simulink model "step_down_chopper"  (R2019b)
settings: Solver=VariableStepAuto  StartTime=0.0  StopTime=0.01  RelTol=1e-3
libraries: powerlib x9, powerlib_meascontrol x1
settings Model: Creator=DELL  LastModifiedBy=DELL

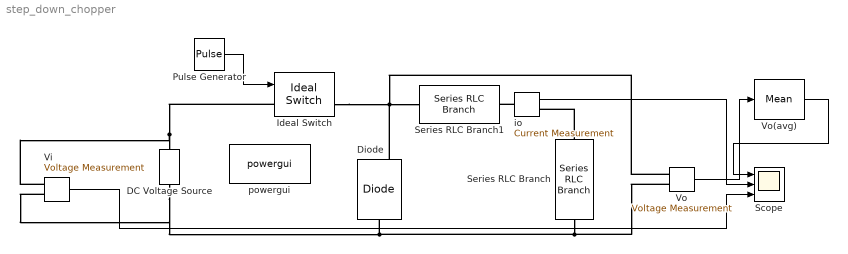
== system step_down_chopper ==
  DC Voltage Source : powerlib/Electrical Sources/DC Voltage Source  Amplitude=200  Measurements=Voltage
      settings: SourceProductName=Simscape Electrical
  Diode : powerlib/Power Electronics/Diode  Ron=0.001  Lon=0  Vf=0.8  IC=0  UseSnubber=0  Rs=500  Cs=250e-9  Measurements=on
      settings: SourceProductName=Simscape Electrical
  Ideal Switch : powerlib/Power Electronics/Ideal Switch  Ron=0.001  Lon=0  IC=0  Rs=1e5  Cs=inf  Measurements=on
      settings: SourceProductName=Simscape Electrical
  Pulse Generator : DiscretePulseGenerator  PulseType=Time based  Period=0.001  PulseWidth=40
  Scope : Scope  NumInputPorts=3
  Series RLC Branch : powerlib/Elements/Series RLC Branch  LConnTagsString=__new0  RConnTagsString=__new0  BranchType=R  Resistance=10  Inductance=1e-3  SetiL0=off  InitialCurrent=0  Capacitance=1e-6  Setx0=off  InitialVoltage=0  Measurements=None
      settings: SourceProductName=Simscape Electrical
  Series RLC Branch1 : powerlib/Elements/Series RLC Branch  LConnTagsString=__new0  RConnTagsString=__new0  BranchType=L  Resistance=1  Inductance=5e-3  SetiL0=off  InitialCurrent=0  Capacitance=1e-6  Setx0=off  InitialVoltage=0  Measurements=None
      settings: SourceProductName=Simscape Electrical
  Vi : powerlib/Measurements/Voltage Measurement  PhasorSimulation=off  OutputType=Complex  PSBequivalent=0
      settings: SourceProductName=Simscape Electrical
  Vo : powerlib/Measurements/Voltage Measurement  PhasorSimulation=off  OutputType=Complex  PSBequivalent=0
      settings: SourceProductName=Simscape Electrical
  Vo(avg) : powerlib_meascontrol/Measurements/Mean  Freq=1000  Vinit=0  Ts=0
      settings: SourceProductName=Simscape Electrical
  io : powerlib/Measurements/Current Measurement  PhasorSimulation=off  OutputType=Complex  PSBequivalent=0
      settings: SourceProductName=Simscape Electrical
  powergui : powerlib/powergui  Priority=1  SimulationMode=Continuous  SampleTime=50e-6  frequency=60  Iterations=50  frequencyindice=0  Pbase=100e6  ErrMax=1e-4  UnitsV=kV  UnitsW=MW  buscounter=0  FunctionMessages=off  echomessages=off  EnableUseOfTLC=off  CurrentSourceSwitches=off  DisableSnubberDevices=off  DisableRonSwitches=off  DisableVfSwitches=off  DisplayEquations=off  AutomaticDiscreteSolvers=off  SolverType=Tustin/Backward Euler (TBE)  Interpol=off  ExternalGateDelay=off  methode=off  Ts=100  x0status=blocks  SPID=on  SwTol=0  HookPort=off  NonlinearTolerance=1e-4  nMaxIteration=100  ContinueOnMaxIteration=off  RestoreLinks=warning  ResistiveCurrentMeasurement=off  Frange=[0:2:500]  Ylog=off  Xlog=on  ShowGrid=off  save=off  variable=ZData  structure=0  ZoomFFT=off  StartTime=0.0  cycles=1  DisplayStyle=1  fundamental=60  FreqAxis=off  MaxFrequency=1000  frequencyindicesteady=1  RmsSteady=1  display=off
      settings: SourceProductName=Simscape Electrical
  wires:
  Pulse Generator/1 -> Ideal Switch/1
  io/1 -> Scope/2
  Vi/1 -> Scope/3
  Vo/1 -> Vo(avg)/1
  Vo(avg)/1 -> Scope/1
  connections:
  Ideal Switch/RConn1 -- Series RLC Branch1/LConn1 -- Vo/LConn1 -- Diode/RConn1
  Ideal Switch/LConn1 -- Vi/LConn1 -- DC Voltage Source/RConn1
  Series RLC Branch/LConn1 -- io/RConn1
  Series RLC Branch/RConn1 -- Diode/LConn1 -- Vi/LConn2 -- DC Voltage Source/LConn1 -- Vo/LConn2
  io/LConn1 -- Series RLC Branch1/RConn1
